simulink model "adim1_basit_antispoofing"  (R2026a)
settings: Solver=FixedStepDiscrete  StopTime=0.006  FixedStep=1/5e6
libraries: simulink x1
settings Model: Creator=ranay  LastModifiedBy=ranay

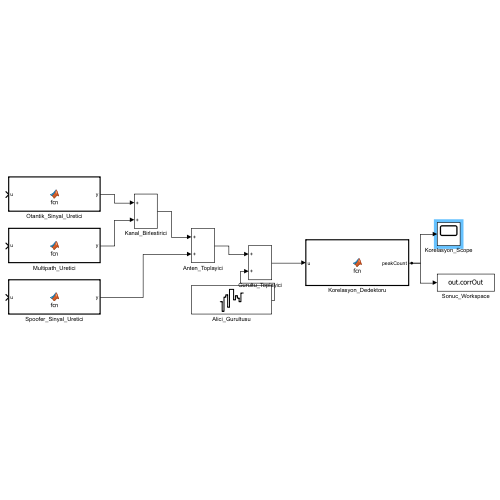
[thumbnail: Simulink's stored preview of the top-level diagram]
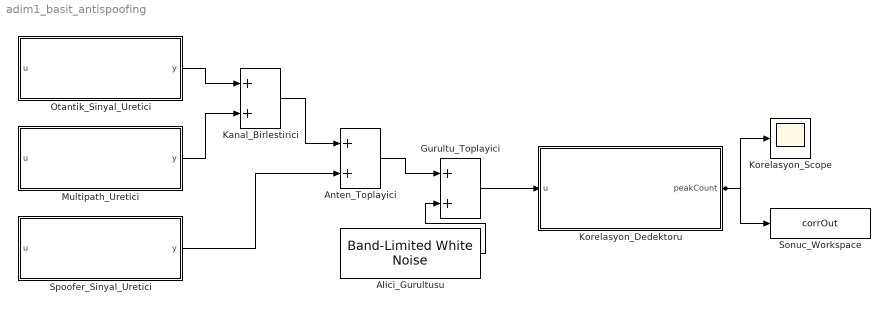
== system adim1_basit_antispoofing ==
  Alici_Gurultusu : simulink/Sources/Band-Limited White Noise  Cov=0  Ts=1/5e6  seed=[23341]
  Anten_Toplayici : Sum
  Gurultu_Toplayici : Sum
  Kanal_Birlestirici : Sum
  Korelasyon_Dedektoru : MATLAB Function  TreatAsAtomicUnit=on
  Korelasyon_Scope : Scope
      settings: ActiveDisplayYMinimum=-0.37499999999999989  ActiveDisplayYMaximum=3.375
  Multipath_Uretici : MATLAB Function  TreatAsAtomicUnit=on
  Otantik_Sinyal_Uretici : MATLAB Function  TreatAsAtomicUnit=on
  Sonuc_Workspace : ToWorkspace  VariableName=corrOut  SaveFormat=Timeseries  SampleTime=-1
  Spoofer_Sinyal_Uretici : MATLAB Function  TreatAsAtomicUnit=on
  wires:
  Otantik_Sinyal_Uretici/1(y) -> Kanal_Birlestirici/1
  Multipath_Uretici/1(y) -> Kanal_Birlestirici/2
  Kanal_Birlestirici/1 -> Anten_Toplayici/1
  Spoofer_Sinyal_Uretici/1(y) -> Anten_Toplayici/2
  Anten_Toplayici/1 -> Gurultu_Toplayici/1
  Alici_Gurultusu/1 -> Gurultu_Toplayici/2
  Gurultu_Toplayici/1 -> Korelasyon_Dedektoru/1(u)
  Korelasyon_Dedektoru/1(peakCount) -> Korelasyon_Scope/1, Sonuc_Workspace/1

== matlab function adim1_basit_antispoofing/Otantik_Sinyal_Uretici ==
  data: u input; y output
function y = fcn(u)
%#codegen
persistent phase t
if isempty(phase); phase = 300; end
if isempty(t); t = 0; end
Fs = 5e6; f_IF = 1.25e6; doppler = 1500; atmos_delay = 0.5;
ca = generate_ca_code(7);
idx = mod(floor(phase + atmos_delay), 1023) + 1;
baseband = ca(idx);
y = baseband * cos(2 * pi * (f_IF + doppler) * t);
phase = phase + 1.023e6/Fs;
t = t + 1/Fs;
end

== matlab function adim1_basit_antispoofing/Spoofer_Sinyal_Uretici ==
  data: u input; y output
function y = fcn(u)
%#codegen
persistent phase t genlik drift
if isempty(phase); phase = 300; end
if isempty(t); t = 0; end
if isempty(genlik); genlik = 1.0; end
if isempty(drift); drift = 0; end
Fs = 5e6; f_IF = 1.25e6; doppler = 1500; atmos_delay = 0.5;
ca = generate_ca_code(7);
drift = drift + 0.002;
idx = mod(floor(phase + atmos_delay + drift), 1023) + 1;
baseband = ca(idx);
genlik = min(genlik + 0.0001, 2.0);
y = genlik * baseband * cos(2 * pi * (f_IF + doppler) * t);
phase = phase + 1.023e6/Fs;
t = t + 1/Fs;
end

== matlab function adim1_basit_antispoofing/Korelasyon_Dedektoru ==
  data: u input; peakCount output
function peakCount = fcn(u)
%#codegen
coder.extrinsic('run_simulink_correlation');
persistent buf count lastPeaks
if isempty(buf); buf = zeros(1, 10000); end
if isempty(count); count = 1; end
if isempty(lastPeaks); lastPeaks = 0; end
buf(count) = u;
count = count + 1;
if count > 10000
    count = 1;
    tempPeaks = 0;
    tempPeaks = run_simulink_correlation(buf);
    lastPeaks = tempPeaks;
end
peakCount = lastPeaks;
end

== matlab function adim1_basit_antispoofing/Multipath_Uretici ==
  data: u input; y output
function y = fcn(u)
%#codegen
persistent phase t
if isempty(phase); phase = 302; end
if isempty(t); t = 0; end
Fs = 5e6; f_IF = 1.25e6; doppler = 1500; atmos_delay = 0.5;
ca = generate_ca_code(7);
idx = mod(floor(phase + atmos_delay), 1023) + 1;
baseband = ca(idx);
y = 0.4 * baseband * cos(2 * pi * (f_IF + doppler) * t);
phase = phase + 1.023e6/Fs;
t = t + 1/Fs;
end
